simulink model "mars_rover_cam"  (R2023a)
settings: Solver=ode23t  StartTime=0.0  StopTime=120  FixedStep=1e-2  MaxStep=0.1  RelTol=1e-3  AbsTol=1e-3  EnableMultiTasking=on
StartFcn:
  | mars_rover_sim_callback
model workspace (MATLAB code in the model file):
  | addpath("mars_rover_helpers");
  | % Load Rover Arm model for IK
  | mdlpath = ['mars_rover_data',filesep,'mars_rover_arm'];
  | load_system(mdlpath);
  | 
  | imdata = zeros(3,3,3);
  | 
  | % Temp
  | Kp_steer = 1;
  | Ki_steer = 1;
  | Kd_steer = 1;
  | 
  | Kp = 1;
  | Ki = 1;
  | Kd = 1;
values from neighbouring files (symbols this model uses):
  mapData = false(197,200)    [mars_rover_params.m]    (also in mars_rover_startup.m)
undefined symbols (not defined in the file or in its folder): cameraData, Rover, roverPath, Terrain, X, Y, Z
libraries: sm_lib x36, nesl_utility x19, robotcorelib x1, simulink_extras x1
(part 2 of 2)

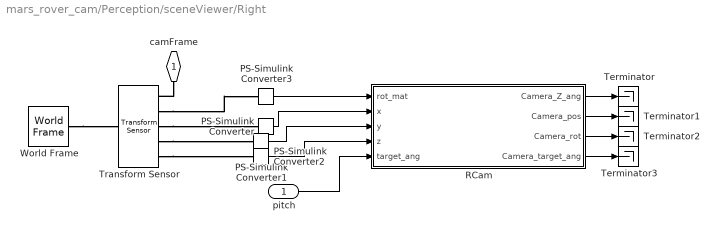
== system mars_rover_cam/Perception/sceneViewer/Right ==
  pitch : Inport
  PS-Simulink Converter{,1..3} (4 alike) : nesl_utility/PS-Simulink Converter  PhysicalDomain=network_engine_domain  SubClassName=ps_output  LeftPortType=input  RightPortType=output  PseudoPeriodic=off  Frequencies=[]  VectorFormat=inherit  Unit=inherit  AffineConversion=off
  RCam : MATLAB Function  TreatAsAtomicUnit=on
  Terminator{,1..3} (4 alike) : Terminator
  Transform Sensor : sm_lib/Frames and Transforms/Transform Sensor  MeasurementFrame=World  RotationSequence=XYX  SenseAngle=off  SenseAxis=off  SenseQ=off  SenseR=on  SenseRotationSequence=off  SenseOmegaX=off  SenseOmegaY=off  SenseOmegaZ=off  SenseQDot=off  SenseRDot=off  SenseRotationSequenceDot=off  SenseAlphaX=off  SenseAlphaY=off  SenseAlphaZ=off  SenseQDDot=off  SenseRDDot=off  SenseX=on  SenseY=on  SenseZ=on  SenseRad=off  SenseAzim=off  SenseDist=off  SenseInc=off  SenseXDot=off  SenseYDot=off  SenseZDot=off  SenseRadDot=off  SenseAzimDot=off  SenseDistDot=off  SenseIncDot=off  SenseXDDot=off  SenseYDDot=off  SenseZDDot=off  SenseRadDDot=off  SenseAzimDDot=off  SenseDistDDot=off  SenseIncDDot=off
  World Frame : sm_lib/Frames and Transforms/World Frame
  camFrame : PMIOPort  Side=Right
  wires:
  RCam/4(Camera_target_ang) -> Terminator3/1
  RCam/3(Camera_rot) -> Terminator2/1
  RCam/1(Camera_Z_ang) -> Terminator/1
  PS-Simulink Converter2/1 -> RCam/4(z)
  PS-Simulink Converter3/1 -> RCam/1(rot_mat)
  PS-Simulink Converter/1 -> RCam/2(x)
  pitch/1 -> RCam/5(target_ang)
  PS-Simulink Converter1/1 -> RCam/3(y)
  RCam/2(Camera_pos) -> Terminator1/1
  connections:
  camFrame/RConn1 -- Transform Sensor/RConn1
  Transform Sensor/RConn2 -- PS-Simulink Converter3/LConn1
  Transform Sensor/RConn3 -- PS-Simulink Converter/LConn1
  Transform Sensor/RConn4 -- PS-Simulink Converter1/LConn1
  World Frame/RConn1 -- Transform Sensor/LConn1
  Transform Sensor/RConn5 -- PS-Simulink Converter2/LConn1

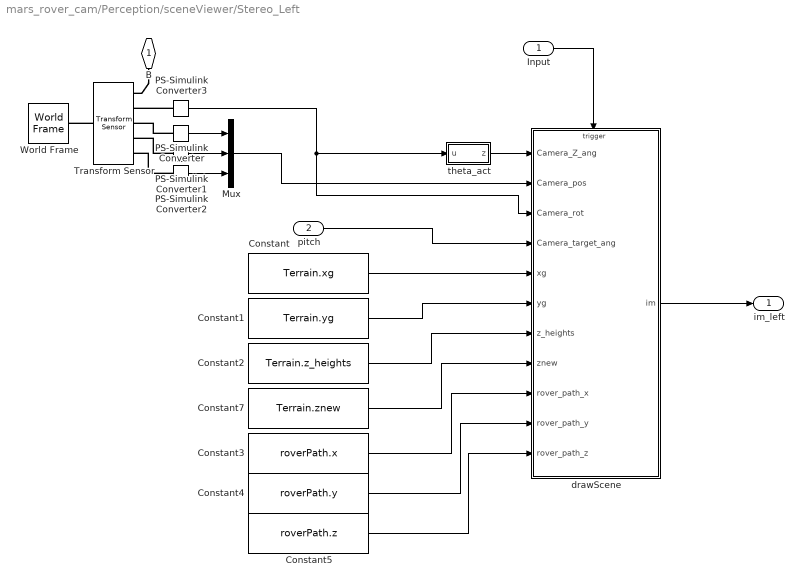
== system mars_rover_cam/Perception/sceneViewer/Stereo_Left ==
  Input : Inport
  pitch : Inport  Port=2
  Constant : Constant  Value=Terrain.xg
  Constant1 : Constant  Value=Terrain.yg
  Constant2 : Constant  Value=Terrain.z_heights
  Constant3 : Constant  Value=roverPath.x
  Constant4 : Constant  Value=roverPath.y
  Constant5 : Constant  Value=roverPath.z
  Constant7 : Constant  Value=Terrain.znew
  Mux : Mux  Inputs=3
  PS-Simulink Converter{,1..3} (4 alike) : nesl_utility/PS-Simulink Converter  PhysicalDomain=network_engine_domain  SubClassName=ps_output  LeftPortType=input  RightPortType=output  PseudoPeriodic=off  Frequencies=[]  VectorFormat=inherit  Unit=inherit  AffineConversion=off
  Transform Sensor : sm_lib/Frames and Transforms/Transform Sensor  MeasurementFrame=World  RotationSequence=XYX  SenseAngle=off  SenseAxis=off  SenseQ=off  SenseR=on  SenseRotationSequence=off  SenseOmegaX=off  SenseOmegaY=off  SenseOmegaZ=off  SenseQDot=off  SenseRDot=off  SenseRotationSequenceDot=off  SenseAlphaX=off  SenseAlphaY=off  SenseAlphaZ=off  SenseQDDot=off  SenseRDDot=off  SenseX=on  SenseY=on  SenseZ=on  SenseRad=off  SenseAzim=off  SenseDist=off  SenseInc=off  SenseXDot=off  SenseYDot=off  SenseZDot=off  SenseRadDot=off  SenseAzimDot=off  SenseDistDot=off  SenseIncDot=off  SenseXDDot=off  SenseYDDot=off  SenseZDDot=off  SenseRadDDot=off  SenseAzimDDot=off  SenseDistDDot=off  SenseIncDDot=off
  World Frame : sm_lib/Frames and Transforms/World Frame
  drawScene : Subsystem
  theta_act : MATLAB Function  TreatAsAtomicUnit=on
  B : PMIOPort  Side=Left
  im_left : Outport
  wires:
  PS-Simulink Converter2/1 -> Mux/3
  Mux/1 -> drawScene/2(Camera_pos)
  PS-Simulink Converter/1 -> Mux/1
  PS-Simulink Converter3/1 -> drawScene/3(Camera_rot), theta_act/1(u)
  PS-Simulink Converter1/1 -> Mux/2
  theta_act/1(z) -> drawScene/1(Camera_Z_ang)
  pitch/1 -> drawScene/4(Camera_target_ang)
  Constant/1 -> drawScene/5(xg)
  Constant1/1 -> drawScene/6(yg)
  Constant2/1 -> drawScene/7(z_heights)
  Constant7/1 -> drawScene/8(znew)
  Constant3/1 -> drawScene/9(rover_path_x)
  Constant4/1 -> drawScene/10(rover_path_y)
  Constant5/1 -> drawScene/11(rover_path_z)
  drawScene/1(im) -> im_left/1
  Input/1 -> drawScene/Trigger
  connections:
  PS-Simulink Converter3/LConn1 -- Transform Sensor/RConn2
  PS-Simulink Converter2/LConn1 -- Transform Sensor/RConn5
  Transform Sensor/LConn1 -- World Frame/RConn1
  PS-Simulink Converter/LConn1 -- Transform Sensor/RConn3
  PS-Simulink Converter1/LConn1 -- Transform Sensor/RConn4
  B/RConn1 -- Transform Sensor/RConn1

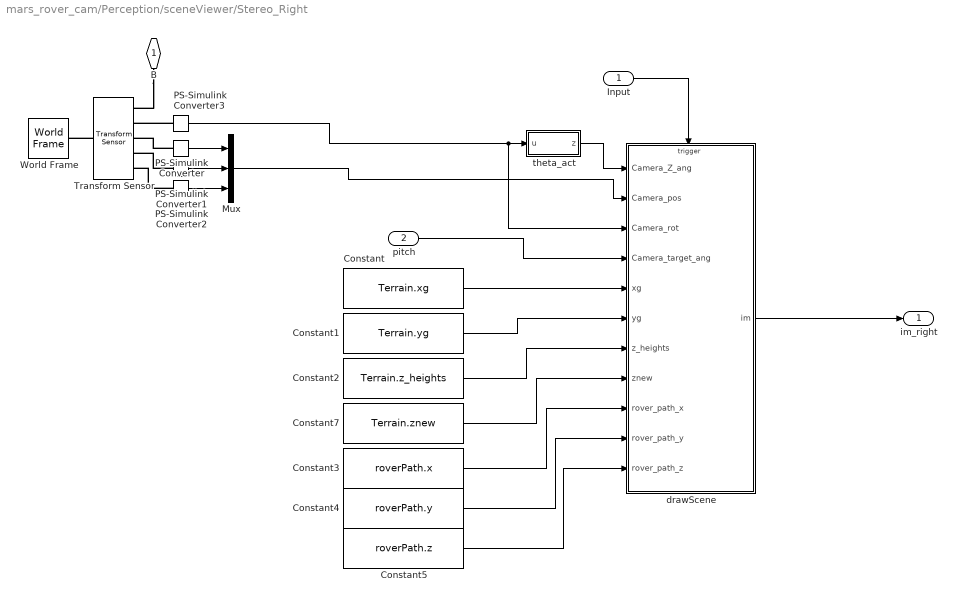
== system mars_rover_cam/Perception/sceneViewer/Stereo_Right ==
  Input : Inport
  pitch : Inport  Port=2
  Constant : Constant  Value=Terrain.xg
  Constant1 : Constant  Value=Terrain.yg
  Constant2 : Constant  Value=Terrain.z_heights
  Constant3 : Constant  Value=roverPath.x
  Constant4 : Constant  Value=roverPath.y
  Constant5 : Constant  Value=roverPath.z
  Constant7 : Constant  Value=Terrain.znew
  Mux : Mux  Inputs=3
  PS-Simulink Converter{,1..3} (4 alike) : nesl_utility/PS-Simulink Converter  PhysicalDomain=network_engine_domain  SubClassName=ps_output  LeftPortType=input  RightPortType=output  PseudoPeriodic=off  Frequencies=[]  VectorFormat=inherit  Unit=inherit  AffineConversion=off
  Transform Sensor : sm_lib/Frames and Transforms/Transform Sensor  MeasurementFrame=World  RotationSequence=XYX  SenseAngle=off  SenseAxis=off  SenseQ=off  SenseR=on  SenseRotationSequence=off  SenseOmegaX=off  SenseOmegaY=off  SenseOmegaZ=off  SenseQDot=off  SenseRDot=off  SenseRotationSequenceDot=off  SenseAlphaX=off  SenseAlphaY=off  SenseAlphaZ=off  SenseQDDot=off  SenseRDDot=off  SenseX=on  SenseY=on  SenseZ=on  SenseRad=off  SenseAzim=off  SenseDist=off  SenseInc=off  SenseXDot=off  SenseYDot=off  SenseZDot=off  SenseRadDot=off  SenseAzimDot=off  SenseDistDot=off  SenseIncDot=off  SenseXDDot=off  SenseYDDot=off  SenseZDDot=off  SenseRadDDot=off  SenseAzimDDot=off  SenseDistDDot=off  SenseIncDDot=off
  World Frame : sm_lib/Frames and Transforms/World Frame
  drawScene : Subsystem
  theta_act : MATLAB Function  TreatAsAtomicUnit=on
  B : PMIOPort  Side=Left
  im_right : Outport
  wires:
  PS-Simulink Converter1/1 -> Mux/2
  PS-Simulink Converter3/1 -> theta_act/1(u), drawScene/3(Camera_rot)
  PS-Simulink Converter/1 -> Mux/1
  Mux/1 -> drawScene/2(Camera_pos)
  PS-Simulink Converter2/1 -> Mux/3
  theta_act/1(z) -> drawScene/1(Camera_Z_ang)
  pitch/1 -> drawScene/4(Camera_target_ang)
  Constant/1 -> drawScene/5(xg)
  Constant1/1 -> drawScene/6(yg)
  Constant2/1 -> drawScene/7(z_heights)
  Constant7/1 -> drawScene/8(znew)
  Constant3/1 -> drawScene/9(rover_path_x)
  Constant4/1 -> drawScene/10(rover_path_y)
  Constant5/1 -> drawScene/11(rover_path_z)
  drawScene/1(im) -> im_right/1
  Input/1 -> drawScene/Trigger
  connections:
  B/RConn1 -- Transform Sensor/RConn1
  PS-Simulink Converter1/LConn1 -- Transform Sensor/RConn4
  PS-Simulink Converter/LConn1 -- Transform Sensor/RConn3
  Transform Sensor/LConn1 -- World Frame/RConn1
  PS-Simulink Converter2/LConn1 -- Transform Sensor/RConn5
  PS-Simulink Converter3/LConn1 -- Transform Sensor/RConn2

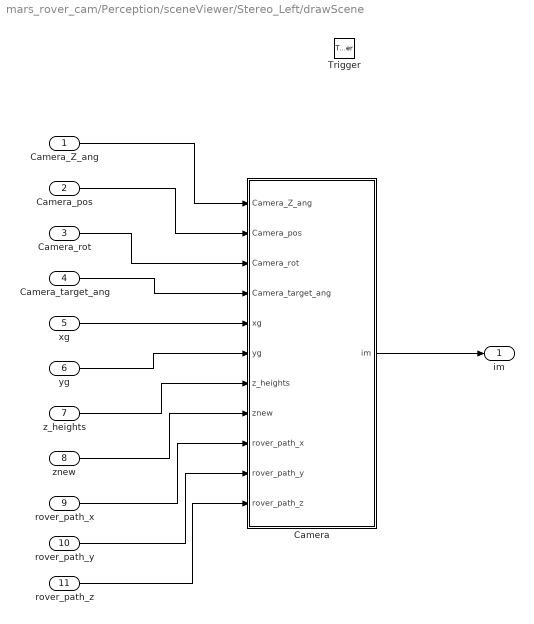
== system mars_rover_cam/Perception/sceneViewer/Stereo_Left/drawScene ==
  Camera_Z_ang : Inport
  Camera_pos : Inport  Port=2
  Camera_rot : Inport  Port=3
  Camera_target_ang : Inport  Port=4
  xg : Inport  Port=5
  yg : Inport  Port=6
  z_heights : Inport  Port=7
  znew : Inport  Port=8
  rover_path_x : Inport  Port=9
  rover_path_y : Inport  Port=10
  rover_path_z : Inport  Port=11
  Trigger : TriggerPort  VariantControl=(inherit)  InitialTriggerSignalState=negative  PortDimensions=1
  Camera : MATLAB Function  TreatAsAtomicUnit=on
  im : Outport
  wires:
  Camera/1(im) -> im/1
  rover_path_x/1 -> Camera/9(rover_path_x)
  Camera_Z_ang/1 -> Camera/1(Camera_Z_ang)
  rover_path_z/1 -> Camera/11(rover_path_z)
  z_heights/1 -> Camera/7(z_heights)
  xg/1 -> Camera/5(xg)
  znew/1 -> Camera/8(znew)
  rover_path_y/1 -> Camera/10(rover_path_y)
  yg/1 -> Camera/6(yg)
  Camera_pos/1 -> Camera/2(Camera_pos)
  Camera_target_ang/1 -> Camera/4(Camera_target_ang)
  Camera_rot/1 -> Camera/3(Camera_rot)

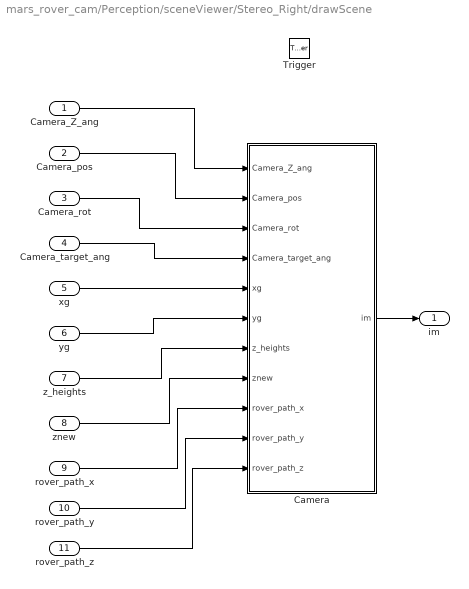
== system mars_rover_cam/Perception/sceneViewer/Stereo_Right/drawScene ==
  Camera_Z_ang : Inport
  Camera_pos : Inport  Port=2
  Camera_rot : Inport  Port=3
  Camera_target_ang : Inport  Port=4
  xg : Inport  Port=5
  yg : Inport  Port=6
  z_heights : Inport  Port=7
  znew : Inport  Port=8
  rover_path_x : Inport  Port=9
  rover_path_y : Inport  Port=10
  rover_path_z : Inport  Port=11
  Trigger : TriggerPort  VariantControl=(inherit)  InitialTriggerSignalState=negative  PortDimensions=1
  Camera : MATLAB Function  TreatAsAtomicUnit=on
  im : Outport
  wires:
  Camera/1(im) -> im/1
  Camera_pos/1 -> Camera/2(Camera_pos)
  rover_path_z/1 -> Camera/11(rover_path_z)
  Camera_target_ang/1 -> Camera/4(Camera_target_ang)
  rover_path_y/1 -> Camera/10(rover_path_y)
  znew/1 -> Camera/8(znew)
  z_heights/1 -> Camera/7(z_heights)
  xg/1 -> Camera/5(xg)
  rover_path_x/1 -> Camera/9(rover_path_x)
  yg/1 -> Camera/6(yg)
  Camera_Z_ang/1 -> Camera/1(Camera_Z_ang)
  Camera_rot/1 -> Camera/3(Camera_rot)

== matlab function mars_rover_cam/Perception/sceneViewer/Stereo_Left/theta_act ==
  data: u input; z output
function z  = fcn(u)
out = rotm2eul(u);
z = out(1);
% y = out(2);
%x = out(3);
end

== matlab function mars_rover_cam/Perception/sceneViewer/Stereo_Right/drawScene/Camera ==
  settings: sampleTime=0.1
  data: Camera_Z_ang input; Camera_pos input; Camera_rot input; Camera_target_ang input; xg input; yg input; z_heights input; znew input; rover_path_x input; rover_path_y input; rover_path_z input; im output
function im = fcn(Camera_Z_ang,...
    Camera_pos,...
    Camera_rot,...
    Camera_target_ang,...
    xg,yg,z_heights,znew,...
    rover_path_x,rover_path_y,rover_path_z)
im = uint8(zeros(420,560,3));
coder.extrinsic('axes')
coder.extrinsic('figure')
coder.extrinsic('plotSurfaceForCamera')
coder.extrinsic('getframe')
coder.extrinsic('moveCamera');
coder.extrinsic('getfield');
coder.extrinsic('print');
coder.extrinsic('frame2im');
coder.extrinsic('imresize');
coder.extrinsic('imshow');

persistent  surface_ax fig ;

if isempty(surface_ax)

    % Plot the Surface plot in MATLAB.
    fh = findobj( 'Type', 'Figure', 'Name', 'RightNavCam ');
    close(fh);
    fig = figure(22);%figure('Name','LeftNavCam');
    set(fig,'Name','RightNavCam');
    set(fig, 'Visible', 'off');
    surface_ax = axes(fig,'XLim',[min(xg) max(xg)],'YLim',[min(yg) max(yg)],'ZLim',[0 8]);
    plotSurfaceForCamera(surface_ax,xg,yg,z_heights,znew);
end

moveCamera_R(surface_ax,Camera_Z_ang,Camera_pos,Camera_rot,Camera_target_ang);
pause(0.005);
frame = getframe(surface_ax);
RGB = frame2im(frame);
im = imresize(RGB,[420 560]);

end

== matlab function mars_rover_cam/Perception/sceneViewer/Stereo_Right/theta_act ==
  data: u input; z output
function z  = fcn(u)
out = rotm2eul(u);
z = out(1);
% y = out(2);
%x = out(3);
end

== matlab function mars_rover_cam/Perception/MLFB ==
  settings: updateMethod=DISCRETE  sampleTime=Rover.detection_sample_time
  data: image input; bboxes output size=[500 4]; thresholdVal parameter; roi parameter
function bboxes  = objectDetector(image,thresholdVal, roi)
isSim = coder.target('sfun');
simSupported = false;
useExtrinsic = isSim && ~simSupported;
if all(roi(:)==0)
    [bboxes, ~] = deep.blocks.internal.objectDetector(image, 'rockDetectorDL.mat', true, {'Threshold', thresholdVal, 'SelectStrongest', false}, {}, 500, true, false, true);
else
    [bboxes, ~] = deep.blocks.internal.objectDetector(image, 'rockDetectorDL.mat', true, {roi,'Threshold', thresholdVal, 'SelectStrongest', false}, {}, 500, true, false, true);
end

== matlab function mars_rover_cam/Perception/depthEstimation ==
  settings: updateMethod=DISCRETE  sampleTime=Rover.detection_sample_time
  data: in_bboxes input; I_left input; I_right input; im_out output; obstacleWorldXYZ output size=[700 4] [..20000]; rover_translation input; rover_orientation input; cam_base_angle input; cam_target_angle input; obstacleDistance output size=[1 700]
function [im_out,obstacleWorldXYZ,obstacleDistance] = fcn(in_bboxes,I_left,I_right,rover_translation,rover_orientation,cam_base_angle,cam_target_angle)

im_out = uint8(zeros(420,560,3));
obstacleWorldXYZ = zeros(500,3);
obstacleDistance = zeros(1,500);
coder.extrinsic("mars_rover_stereo_vision");

if ~isempty(in_bboxes)
    [im_out, obstacleWorldXYZ, obstacleDistance] = mars_rover_stereo_vision(I_left,I_right,in_bboxes,rover_translation,rover_orientation,cam_base_angle,cam_target_angle);
else
    im_out = I_left;
end


end

== matlab function mars_rover_cam/Perception/rocksOnPath ==
  settings: updateMethod=DISCRETE  sampleTime=Rover.detection_sample_time
  data: obstacleWorldXYZ input; obstacleDistance input; roverPath input; rocksOnPath output; rePlanFlag output; mapData input
function [rocksOnPath ,rePlanFlag]= fcn(obstacleWorldXYZ,obstacleDistance,roverPath,mapData)

% Create a circle with radius of 0.8 m and center at obstacleLocation

rocksOnPath = zeros(100,3);
rocks_path = zeros(100,3);
rePlanFlag = 0;
% roverPath = [roverPath_x roverPath_y];
k = 1;
map = binaryOccupancyMap(mapData,'resolution',5);

if any(obstacleDistance(:))

    for i = 1:size(obstacleWorldXYZ,1)

        if obstacleDistance(i) <= 3.5 

            x_rock = obstacleWorldXYZ(i,1);
            y_rock = obstacleWorldXYZ(i,2);
          
            for j = 1:size(roverPath,1)

                x_path = roverPath(j,1);
                y_path = roverPath(j,2);

                dist = sqrt((x_path-x_rock)^2 + (y_path-y_rock)^2);
                 if dist <= 1.4
                    rocks_path(k,:) = obstacleWorldXYZ(i,:);
                    rePlanFlag = 1;
                    k = k+1;
                end
              
            end
        end

    end
end

rocks_path = unique(rocks_path,'rows');

for r = 1:size(rocks_path,1)

    rocksOnPath(r,:) = rocks_path(r,:);

end


end

== matlab function mars_rover_cam/Perception/sceneViewer/Left/LCam ==
  settings: updateMethod=DISCRETE  sampleTime=0.8
  data: rot_mat input; Camera_Z_ang output; Camera_pos output; Camera_rot output; Camera_target_ang output; x input; y input; z input; target_ang input
function [Camera_Z_ang, Camera_pos, Camera_rot, Camera_target_ang]= fcn(rot_mat,x,y,z,target_ang)

out = rotm2eul(rot_mat);
Camera_Z_ang = out(1);
Camera_pos = [x y z];
Camera_rot = rot_mat;
Camera_target_ang = target_ang;
end

== matlab function mars_rover_cam/Perception/sceneViewer/Right/RCam ==
  settings: updateMethod=DISCRETE  sampleTime=0.8
  data: rot_mat input; Camera_Z_ang output; Camera_pos output; Camera_rot output; Camera_target_ang output; x input; y input; z input; target_ang input
function [Camera_Z_ang, Camera_pos, Camera_rot, Camera_target_ang]= fcn(rot_mat,x,y,z,target_ang)

out = rotm2eul(rot_mat);
Camera_Z_ang = out(1);
Camera_pos = [x y z];
Camera_rot = rot_mat;
Camera_target_ang = target_ang;
end

== matlab function mars_rover_cam/Perception/sceneViewer/Stereo_Left/drawScene/Camera ==
  settings: sampleTime=0.1
  data: Camera_Z_ang input; Camera_pos input; Camera_rot input; Camera_target_ang input; xg input; yg input; z_heights input; znew input; rover_path_x input; rover_path_y input; rover_path_z input; im output
 function im = fcn(Camera_Z_ang,...
                         Camera_pos,...
                         Camera_rot,...
                         Camera_target_ang,...
                         xg,yg,z_heights,znew,...
                         rover_path_x,rover_path_y,rover_path_z)
im = uint8(zeros(420,560,3));
coder.extrinsic('axes')
coder.extrinsic('figure')
coder.extrinsic('plotSurfaceForCamera')
coder.extrinsic('getframe')
coder.extrinsic('moveCamera');
coder.extrinsic('getfield');
coder.extrinsic('print');
coder.extrinsic('frame2im');
coder.extrinsic('imresize');
coder.extrinsic('imshow');

persistent  surface_ax  fig ; 

if isempty(surface_ax)
  
    % Plot the Surface plot in MATLAB.
    fh = findobj( 'Type', 'Figure', 'Name', 'LeftNavCam ');
    close(fh);
    fig = figure(21);
    set(fig,'Name','LeftNavCam');       
    set(fig, 'Visible', 'off');
    surface_ax = axes(fig,'XLim',[min(xg) max(xg)],'YLim',[min(yg) max(yg)],'ZLim',[0 8]);    
    plotSurfaceForCamera(surface_ax,xg,yg,z_heights,znew);
end

 moveCamera_L(surface_ax,Camera_Z_ang,Camera_pos,Camera_rot,Camera_target_ang);
 pause(0.005);
 frame = getframe(surface_ax);
 RGB = frame2im(frame);
 im = imresize(RGB,[420 560]);

end
